simulink model "sampleModel1639"  (R2023a)
settings: Solver=VariableStepAuto  StartTime=0.0  StopTime=10.0  RelTol=1e-3
libraries: hdlsllib x3, simulink x1
settings Model: Creator=user1  LastModifiedBy=user1

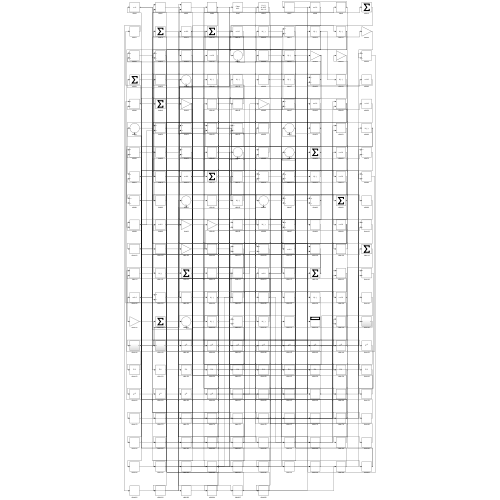
[thumbnail: Simulink's stored preview of the top-level diagram]
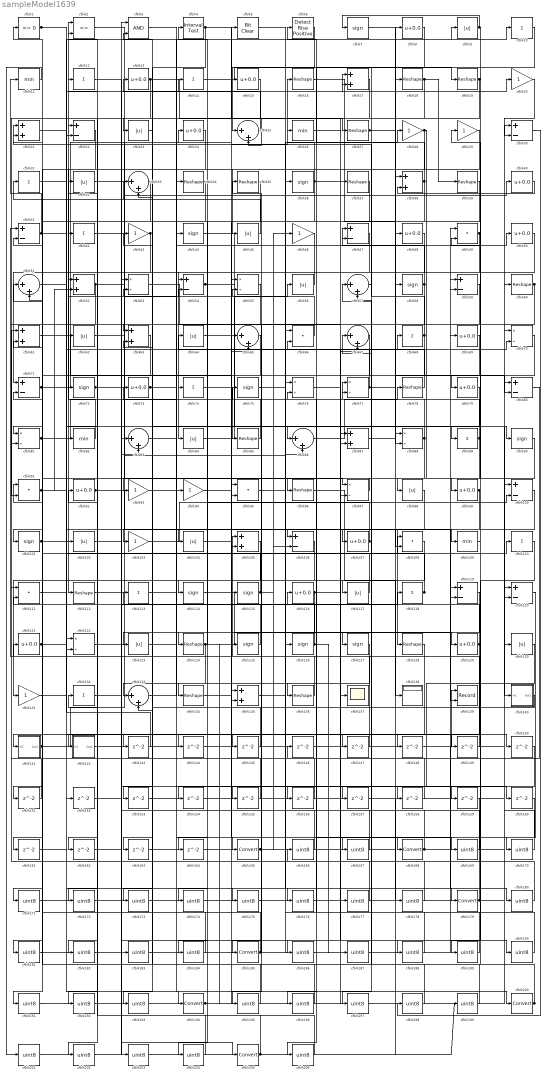
== system sampleModel1639 ==
  cfblk1 : hdlsllib/Logic and Bit Operations/Compare To Zero  relop=<=  OutDataTypeStr=boolean
  cfblk{10,12,14,31,42,68,74,89,110,113,118,132} (12 alike) : Sum  Inputs=+
  cfblk{22,30,41,47,54,59,71,80,100,106,119..120} (12 alike) : Sum  Inputs=+-
  cfblk{7,36,44,58,72,75,90,101,114..115,125..127} (13 alike) : Signum
  cfblk{9,23,32,45,56,62,64,84,98,102,104,117,123,130} (14 alike) : Abs  SaturateOnIntegerOverflow=off
  cfblk{20,28..29,43,46,93..94,103,131} (9 alike) : Gain
  cfblk{17,21,38,52,61,63,87,105,135} (9 alike) : Sum
  cfblk{8,13,15,24,40,48,50,69,73,79,92,99,107,116,121,129} (16 alike) : Bias  Bias=0.0  SaturateOnIntegerOverflow=off
  cfblk{49,66,91,95,108,111} (6 alike) : DotProduct  OutDataTypeStr=Inherit: Inherit via internal rule
  cfblk{11,26,82,109} (4 alike) : MinMax
  cfblk{16,18..19,27,34..35,37,39,60,78,85,96,112,124,128,134,136} (17 alike) : Reshape
  cfblk{53,55,70,76..77,81,88,97,122} (9 alike) : Product  Inputs=*/  RndMeth=Zero  SaturateOnIntegerOverflow=on
  cfblk{25,33,51,57,65,67,83,86,133} (9 alike) : Sum  Inputs=|++
  cfblk137 : Scope
  cfblk138 : Display
  cfblk139 : Record  FileSettingsInternal="{\"entries\":[{\"content\":{\"excelSettings\":{\"content\":{},\"type\":\"Streamout.ExcelSettings\"}},\"type\":\"Streamout.FileSettingStorage\",\"uuid\":\"\"}],\"packageUris\":[\"http:\\/\\/schema.mathworks.com\\/mf0\\/streamout_blocks\\/R2020a\"],\"version\":\"1.0\"}"  Layout=[1 1]  SignalsInternal="{\"entries\":[{\"content\":{\"signals\":[{\"content\":{\"blockPath\":[],\"dimensions\":[1],\"domain\":\"\",\"lineColor\":\"#a2142f\",\"plots\":[1],\"port\":1,\"signalID\":2452,\"signalName\":\"XY Graph:1\"},\"type\":\"RecordBlkView.Signal\",\"uuid\":\"\"},{\"content\":{\"blockPath\":[],\"dimensions\":[1],\"domain\":\"\",\"lineColor\":\"#139fff\",\"plots\":[1],\"port\":2,\"signalID\":2455,\"signalName\":\"XY Graph:2\"},\"type\":\"RecordBlkView.Signal\",\"uuid\":\"\"}]},\"type\":\"RecordBlkView.InputSignals\",\"uuid\":\"\"}],\"packageUris\":[\"http:\\/\\/schema.mathworks.com\\/mf0\\/streamout_blocks\\/R2020a\"],\"version\":\"1.0\"}"  VisualizationBindings="{\"xyplotplugin\":{\"info\":[{\"series\":[{\"bindingParametersList\":[{\"parameter\":\"X-Axis\",\"signalID\":2452,\"signalName\":\"XY Graph:1\"},{\"parameter\":\"Y-Axis\",\"signalID\":2455,\"signalName\":\"XY Graph:2\"}],\"seriesID\":7523}],\"subplotID\":1}]}}"  CompatibilityTag=XY  st=-1
  cfblk140 : Subsystem
      settings: LibrarySourceBlock=|
      | hdlsllib/Ports &
      | Subsystems/Subsystem
  cfblk141 : Subsystem
      settings: LibrarySourceBlock=|
      | hdlsllib/Ports &
      | Subsystems/Subsystem
  cfblk142 : Subsystem
      settings: LibrarySourceBlock=|
      | hdlsllib/Ports &
      | Subsystems/Subsystem
  cfblk{143..164} (22 alike) : Delay  SampleTime=1
  cfblk{165,168,179,185,194,200,205} (7 alike) : DataTypeConversion  SaturateOnIntegerOverflow=off  RndMeth=Floor
  cfblk{166..167,169..178,180..184,186..193,195..199,201..204,206} (35 alike) : DataTypeConversion  OutDataTypeStr=uint8  SaturateOnIntegerOverflow=off  RndMeth=Floor
  cfblk2 : RelationalOperator  Operator=<=  OutDataTypeStr=boolean  InputSameDT=off
  cfblk3 : Logic  AllPortsSameDT=off  OutDataTypeStr=boolean
  cfblk4 : hdlsllib/Logic and Bit Operations/Interval Test  IntervalClosedRight=on  uplimit=0.5  IntervalClosedLeft=on  lowlimit=-0.5  OutDataTypeStr=boolean
  cfblk5 : simulink/Logic and Bit Operations/Bit Clear  iBit=0
      settings: LibrarySourceBlock=|
      | hdlsllib/Logic and Bit
      | Operations/Bit Clear
  cfblk6 : hdlsllib/Logic and Bit Operations/Detect Rise Positive  vinit=0  OutDataTypeStr=boolean
  wires:
  cfblk91/1 -> cfblk52/2, cfblk149/1
  cfblk97/1 -> cfblk96/1
  cfblk136/1 -> cfblk105/1
  cfblk92/1 -> cfblk128/1, cfblk66/1
  cfblk3/1 -> cfblk165/1
  cfblk14/1 -> cfblk19/1
  cfblk114/1 -> cfblk127/1
  cfblk46/1 -> cfblk71/1
  cfblk72/1 -> cfblk68/1, cfblk157/1
  cfblk6/1 -> cfblk25/1
  cfblk2/1 -> cfblk86/1
  cfblk82/1 -> cfblk2/1
  cfblk8/1 -> cfblk117/1
  cfblk18/1 -> cfblk142/1(In1), cfblk39/1, cfblk153/1
  cfblk47/1 -> cfblk84/1
  cfblk107/1 -> cfblk4/1, cfblk167/1
  cfblk122/1 -> cfblk24/1
  cfblk55/1 -> cfblk74/1
  cfblk22/1 -> cfblk112/1
  cfblk69/1 -> cfblk101/1
  cfblk12/1 -> cfblk205/1
  cfblk32/1 -> cfblk97/1
  cfblk124/1 -> cfblk129/1, cfblk14/1, cfblk163/1
  cfblk66/1 -> cfblk22/1
  cfblk140/1(Out1) -> cfblk41/1
  cfblk9/1 -> cfblk99/1, cfblk7/1
  cfblk56/1 -> cfblk54/1
  cfblk71/1 -> cfblk20/1, cfblk9/1
  cfblk86/1 -> cfblk78/1
  cfblk129/1 -> cfblk41/2, cfblk172/1
  cfblk78/1 -> cfblk64/1
  cfblk28/1 -> cfblk98/1, cfblk181/1
  cfblk10/1 -> cfblk136/1
  cfblk52/1 -> cfblk5/1, cfblk151/1
  cfblk109/1 -> cfblk29/1
  cfblk95/1 -> cfblk28/1
  cfblk112/1 -> cfblk40/1
  cfblk84/1 -> cfblk56/1
  cfblk77/1 -> cfblk8/1, cfblk54/2
  cfblk88/1 -> cfblk77/1, cfblk174/1
  cfblk83/1 -> cfblk200/1
  cfblk60/1 -> cfblk114/1, cfblk133/2
  cfblk43/1 -> cfblk72/1, cfblk192/1
  cfblk116/1 -> cfblk70/2, cfblk67/2, cfblk145/1
  cfblk75/1 -> cfblk47/1
  cfblk99/1 -> cfblk139/2, cfblk193/1, cfblk204/1
  cfblk125/1 -> cfblk53/2
  cfblk142/1(Out1) -> cfblk139/1
  cfblk16/1 -> cfblk88/2
  cfblk108/1 -> cfblk131/1
  cfblk113/1 -> cfblk168/1
  cfblk42/1 -> cfblk15/1
  cfblk1/1 -> cfblk122/2, cfblk106/1
  cfblk105/1 -> cfblk124/1
  cfblk61/1 -> cfblk95/2
  cfblk127/1 -> cfblk134/1
  cfblk85/1 -> cfblk43/1
  cfblk133/1 -> cfblk50/1
  cfblk89/1 -> cfblk55/2, cfblk155/1
  cfblk118/1 -> cfblk91/1, cfblk21/2
  cfblk54/1 -> cfblk89/1, cfblk87/2
  cfblk36/1 -> cfblk16/1, cfblk109/1, cfblk105/2
  cfblk141/1(Out1) -> cfblk94/1, cfblk118/1
  cfblk74/1 -> cfblk85/1
  cfblk44/1 -> cfblk140/1(In1)
  cfblk29/1 -> cfblk45/1
  cfblk96/1 -> cfblk138/1
  cfblk131/1 -> cfblk110/1
  cfblk68/1 -> cfblk21/1, cfblk93/1
  cfblk51/1 -> cfblk194/1
  cfblk81/1 -> cfblk34/1, cfblk90/1
  cfblk62/1 -> cfblk44/1
  cfblk23/1 -> cfblk103/1
  cfblk53/1 -> cfblk126/1
  cfblk19/1 -> cfblk42/1, cfblk25/2
  cfblk4/1 -> cfblk27/1, cfblk63/1
  cfblk41/1 -> cfblk11/1, cfblk108/2
  cfblk115/1 -> cfblk73/1, cfblk106/2
  cfblk121/1 -> cfblk108/1, cfblk66/2
  cfblk25/1 -> cfblk13/1
  cfblk63/1 -> cfblk81/1
  cfblk59/1 -> cfblk185/1
  cfblk79/1 -> cfblk123/1
  cfblk87/1 -> cfblk38/1
  cfblk31/1 -> cfblk62/1
  cfblk24/1 -> cfblk82/1
  cfblk135/1 -> cfblk179/1
  cfblk117/1 -> cfblk75/1
  cfblk40/1 -> cfblk38/2
  cfblk58/1 -> cfblk47/2, cfblk91/2
  cfblk101/1 -> cfblk102/1, cfblk17/2
  cfblk134/1 -> cfblk26/1
  cfblk20/1 -> cfblk30/2
  cfblk27/1 -> cfblk80/2, cfblk147/1
  cfblk7/1 -> cfblk79/1
  cfblk70/1 -> cfblk133/1
  cfblk15/1 -> cfblk22/2
  cfblk103/1 -> cfblk100/2
  cfblk126/1 -> cfblk32/1, cfblk187/1
  cfblk34/1 -> cfblk141/1(In1)
  cfblk73/1 -> cfblk17/1, cfblk10/1
  cfblk17/1 -> cfblk23/1
  cfblk38/1 -> cfblk6/1, cfblk97/2
  cfblk45/1 -> cfblk31/1
  cfblk37/1 -> cfblk104/1
  cfblk49/1 -> cfblk107/1, cfblk52/1
  cfblk13/1 -> cfblk37/1, cfblk81/2
  cfblk35/1 -> cfblk143/1
  cfblk143/1 -> cfblk122/1
  cfblk98/1 -> cfblk144/1
  cfblk144/1 -> cfblk100/1
  cfblk145/1 -> cfblk53/1
  cfblk80/1 -> cfblk146/1
  cfblk146/1 -> cfblk70/1
  cfblk147/1 -> cfblk1/1
  cfblk94/1 -> cfblk148/1
  cfblk149/1 -> cfblk95/1
  cfblk5/1 -> cfblk150/1
  cfblk151/1 -> cfblk61/1
  cfblk21/1 -> cfblk152/1
  cfblk153/1 -> cfblk30/1
  cfblk39/1 -> cfblk154/1
  cfblk154/1 -> cfblk49/1
  cfblk155/1 -> cfblk2/2
  cfblk93/1 -> cfblk156/1
  cfblk156/1 -> cfblk71/2
  cfblk130/1 -> cfblk158/1
  cfblk158/1 -> cfblk55/1
  cfblk104/1 -> cfblk159/1
  cfblk123/1 -> cfblk160/1
  cfblk128/1 -> cfblk161/1
  cfblk67/1 -> cfblk162/1
  cfblk163/1 -> cfblk86/2
  cfblk106/1 -> cfblk164/1
  cfblk164/1 -> cfblk88/1
  cfblk165/1 -> cfblk48/1, cfblk46/1
  cfblk159/1 -> cfblk166/1
  cfblk166/1 -> cfblk3/1
  cfblk167/1 -> cfblk3/2
  cfblk168/1 -> cfblk67/1, cfblk60/1
  cfblk64/1 -> cfblk169/1
  cfblk169/1 -> cfblk113/1
  cfblk120/1 -> cfblk170/1
  cfblk170/1 -> cfblk80/1
  cfblk90/1 -> cfblk171/1
  cfblk171/1 -> cfblk120/1
  cfblk172/1 -> cfblk120/2
  cfblk119/1 -> cfblk173/1
  cfblk173/1 -> cfblk115/1
  cfblk174/1 -> cfblk119/1
  cfblk161/1 -> cfblk175/1
  cfblk175/1 -> cfblk119/2
  cfblk111/1 -> cfblk176/1
  cfblk176/1 -> cfblk69/1
  cfblk26/1 -> cfblk177/1
  cfblk177/1 -> cfblk111/1
  cfblk157/1 -> cfblk178/1
  cfblk178/1 -> cfblk111/2
  cfblk179/1 -> cfblk77/2, cfblk121/1
  cfblk148/1 -> cfblk180/1
  cfblk180/1 -> cfblk135/1
  cfblk181/1 -> cfblk135/2
  cfblk33/1 -> cfblk182/1
  cfblk182/1 -> cfblk36/1
  cfblk102/1 -> cfblk183/1
  cfblk183/1 -> cfblk33/1
  cfblk150/1 -> cfblk184/1
  cfblk184/1 -> cfblk33/2
  cfblk185/1 -> cfblk61/2, cfblk137/1, cfblk35/1
  cfblk162/1 -> cfblk186/1
  cfblk186/1 -> cfblk59/1
  cfblk187/1 -> cfblk59/2
  cfblk76/1 -> cfblk188/1
  cfblk188/1 -> cfblk116/1
  cfblk110/1 -> cfblk189/1
  cfblk189/1 -> cfblk76/1
  cfblk152/1 -> cfblk190/1
  cfblk190/1 -> cfblk76/2
  cfblk65/1 -> cfblk191/1
  cfblk191/1 -> cfblk130/1
  cfblk192/1 -> cfblk65/1
  cfblk193/1 -> cfblk65/2
  cfblk194/1 -> cfblk87/1, cfblk125/1
  cfblk100/1 -> cfblk195/1
  cfblk195/1 -> cfblk51/1
  cfblk160/1 -> cfblk196/1
  cfblk196/1 -> cfblk51/2
  cfblk57/1 -> cfblk197/1
  cfblk197/1 -> cfblk18/1
  cfblk30/1 -> cfblk198/1
  cfblk198/1 -> cfblk57/1
  cfblk199/1 -> cfblk57/2
  cfblk200/1 -> cfblk63/2, cfblk49/2
  cfblk11/1 -> cfblk201/1
  cfblk201/1 -> cfblk83/1
  cfblk50/1 -> cfblk202/1
  cfblk202/1 -> cfblk83/2
  cfblk132/1 -> cfblk203/1
  cfblk203/1 -> cfblk58/1
  cfblk204/1 -> cfblk132/1
  cfblk205/1 -> cfblk199/1, cfblk92/1
  cfblk48/1 -> cfblk206/1
  cfblk206/1 -> cfblk12/1

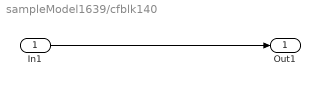
== system sampleModel1639/cfblk140 ==
  In1 : Inport
  Out1 : Outport
  wires:
  In1/1 -> Out1/1

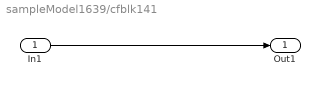
== system sampleModel1639/cfblk141 ==
  In1 : Inport
  Out1 : Outport
  wires:
  In1/1 -> Out1/1

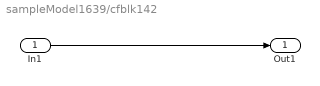
== system sampleModel1639/cfblk142 ==
  In1 : Inport
  Out1 : Outport
  wires:
  In1/1 -> Out1/1
